simulink model "clean_SU_PEREHOD"  (R2021a)
settings: Solver=VariableStepAuto  StartTime=0.0  StopTime=stop  MaxStep=maxdt  MinStep=maxdt/10  RelTol=1e-5
values from neighbouring files (symbols this model uses):
  a_1P = M1U/J1K    (= 0.00153380423814)    [NASTROYKI.m]
  a_2P = M2U/J2K    (= 0.00155623811613)    [NASTROYKI.m]
  a_3P = M3U/J3K    (= 0.00948306595365)    [NASTROYKI.m]
  dt = 5    [NASTROYKI_STAB.m]
  DtR = pi/180    (= 0.0174532925199)    [NASTROYKI.m]    (also in NASTROYKI_STAB.m; NASTROYKI_VSEGO.m)
  g_1P = (M1B+Mmah)/J3K    (= 2.22905525847e-05)    [NASTROYKI.m]
  g_2P = (M2B+Mmah)/J3K    (= 2.22825311943e-05)    [NASTROYKI.m]
  g_3P = (M3B+Mmah)/J3K    (= 2.22905525847e-05)    [NASTROYKI.m]
  J2K = 6837    [NASTROYKI.m]    (also in NASTROYKI_STAB.m; NASTROYKI_VSEGO.m)
  J2M = 2    [NASTROYKI.m]    (also in NASTROYKI_STAB.m; NASTROYKI_VSEGO.m)
  k_1P = 0.5*sqrt((y_0_1P^2)/(2*a_1P^2*RtD^2))    [NASTROYKI.m]
  k_2P = 0.5*sqrt((y_0_2P^2)/(2*a_2P^2*RtD^2))    [NASTROYKI.m]
  k_3P = 0.5*sqrt((y_0_3P^2)/(2*a_3P^2*RtD^2))    [NASTROYKI.m]
  RtD = 1/DtR    (= 57.2957795131)    [NASTROYKI.m]    (also in NASTROYKI_STAB.m; NASTROYKI_VSEGO.m)
  x_0_1P = 0    [NASTROYKI.m]
  x_0_2P = 0    [NASTROYKI.m]
  x_0_3P = 0    [NASTROYKI.m]
  y_0_1P = a_1P*RtD*tmin/2*10    (= 0.00878805094449)    [NASTROYKI.m]
  y_0_2P = a_2P*RtD*tmin/2*10    (= 0.00891658759718)    [NASTROYKI.m]
  y_0_3P = a_3P*RtD*tmin/2*10    (= 0.0543339655989)    [NASTROYKI.m]
undefined symbols (not defined in the file or in its folder): Earth, WGS84
libraries: aerolibanim x4, templibrary x3, aerolibfltsims x2, aerolibtransform2 x1
settings Model: SimulationMode=rapid-accelerator  Creator=vanya  LastModifiedBy=vanya
settings SolverCC: MaxConsecutiveMinStep=50  ShapePreserveControl=EnableAll  ZeroCrossControl=DisableAll  ZeroCrossAlgorithm=Adaptive
settings DebuggingCC: IgnoredZcDiagnostic=none

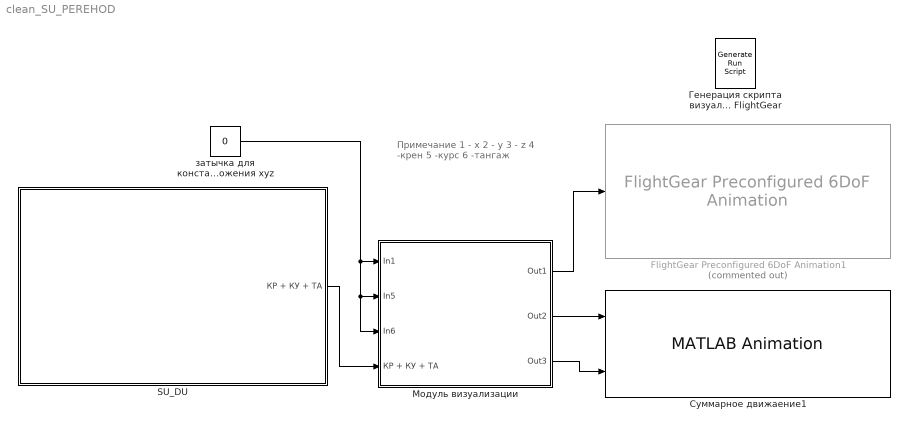
== system clean_SU_PEREHOD ==
  note: Примечание
      | 1 - x
      | 2 - y
      | 3 - z
      | 4 -крен
      | 5 -курс
      | 6 -тангаж
  FlightGear Preconfigured 6DoF Animation1 : aerolibfltsims/FlightGear Preconfigured 6DoF Animation  Commented=on  xFlightGearVersion=v2017.3  DestinationIpAddress=127.0.0.1  DestinationPort=5502  SampleTime=dt  packetVersion=24
  SU_DU : Subsystem
  Генерация скрипта визуализации в FlightGear : aerolibfltsims/Generate Run Script  Architecture=Default  dataFlow=Send  GeometryModelName=14bis  AirportId=KSFO  RunwayId=10L  InitialAltitude=722*100  InitialHeading=113  OffsetDistance=4.72  OffsetAzimuth=0  InstallScenery=off  DisableShaders=off  OriginAddress=127.0.0.1  DestinationPort=5502  OriginPort=5505  LocalAddress=127.0.0.1  OutputFileName=runfg.bat  FlightGearBaseDirectory=C:\Program Files\FlightGear 2020.3
  Модуль визуализации : Subsystem
  Суммарное движаение1 : aerolibanim/MATLAB Animation  Tag=Matlab Animation 6 DOF  Vehicles=1  Geometries='astredwedge.mat'  BoundingBoxCoordinates=[-50,50,-50,50,-50,50]  CameraOffset=[150,-150,-150]  CameraViewAngle=1  SampleTime=0.1  FigurePosition=[1,41,1920,990]
      settings: SourceProductBaseCode=AE
  затычка для константного положения xyz : Constant  Value=0
  wires:
  Модуль визуализации/2(Out2) -> Суммарное движаение1/1
  затычка для константного положения xyz/1 -> Модуль визуализации/3(In6), Модуль визуализации/2(In5), Модуль визуализации/1(In1)
  Модуль визуализации/1(Out1) -> FlightGear Preconfigured 6DoF Animation1/1
  SU_DU/1(КР + КУ + ТА) -> Модуль визуализации/4(КР + КУ + ТА)
  Модуль визуализации/3(Out3) -> Суммарное движаение1/2

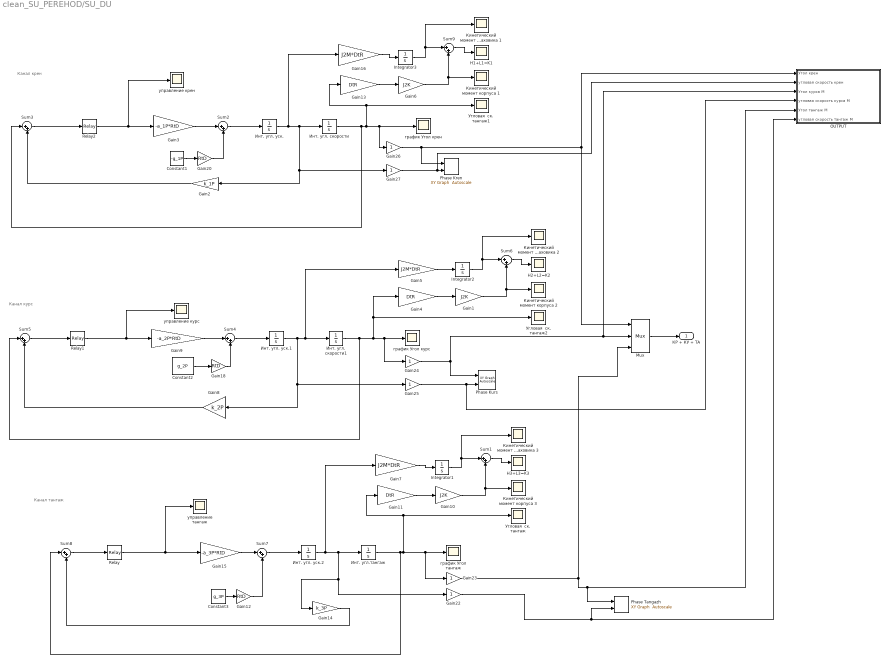
== system clean_SU_PEREHOD/SU_DU ==
  note: Канал крен
  note: Канал курс
  note: Канал тангаж
  " Кинетический момент корпуса 1" : Scope
  " Кинетический момент корпуса 2" : Scope
  " Кинетический момент корпуса 3" : Scope
  Constant1 : Constant  Value=-g_1P
  Constant2 : Constant  Value=g_2P
  Constant3 : Constant  Value=g_3P
  Gain1 : Gain  Gain=J2K
  Gain10 : Gain  Gain=J2K
  Gain11 : Gain  Gain=DtR
  Gain12 : Gain  Gain=RtD
  Gain13 : Gain  Gain=DtR
  Gain14 : Gain  Gain=k_3P
  Gain15 : Gain  Gain=-a_3P*RtD
  Gain16 : Gain  Gain=J2M*DtR
  Gain18 : Gain  Gain=RtD
  Gain2 : Gain  Gain=k_1P
  Gain20 : Gain  Gain=RtD
  Gain{22..27} (6 alike) : Gain
  Gain3 : Gain  Gain=-a_1P*RtD
  Gain4 : Gain  Gain=DtR
  Gain5 : Gain  Gain=J2M*DtR
  Gain6 : Gain  Gain=J2K
  Gain7 : Gain  Gain=J2M*DtR
  Gain8 : Gain  Gain=k_2P
  Gain9 : Gain  Gain=-a_2P*RtD
  H1+L1=K1 : Scope
  H2+L2=K2 : Scope
  H3+L3=K3 : Scope
  Integrator1 : Integrator
  Integrator2 : Integrator
  Integrator3 : Integrator
  Mux : Mux  Inputs=3
  OUTPUT : Subsystem
  Phase Kren : templibrary/XY Graph  Autoscale  xmin=-1  xmax=1  ymin=-1  ymax=1  st=-1
  Phase Kurs : templibrary/XY Graph  Autoscale  xmin=-1  xmax=1  ymin=-1  ymax=1  st=-1
  Phase Tangazh : templibrary/XY Graph  Autoscale  xmin=-1  xmax=1  ymin=-1  ymax=1  st=-1
  Relay : Relay  OnSwitchValue=0  OffSwitchValue=0  OffOutputValue=-1
  Relay1 : Relay  OnSwitchValue=0  OffSwitchValue=0  OffOutputValue=-1
  Relay2 : Relay  OnSwitchValue=0  OffSwitchValue=0  OffOutputValue=-1
  Sum{1..9} (9 alike) : Sum  Inputs=|++
  Инт. угл. скорости : Integrator  InitialCondition=x_0_1P
  Инт. угл. скорости1 : Integrator  InitialCondition=x_0_2P
  Инт. угл. уск. : Integrator  InitialCondition=y_0_1P
  Инт. угл. уск.1 : Integrator  InitialCondition=y_0_2P
  Инт. угл. уск.2 : Integrator  InitialCondition=y_0_3P
  Инт. угл.тангаж : Integrator  InitialCondition=x_0_3P
  Кинетический момент маховика 1 : Scope
  Кинетический момент маховика 2 : Scope
  Кинетический момент маховика 3 : Scope
  Угловая  ск. тангаж : Scope
  Угловая  ск. тангаж1 : Scope
  Угловая  ск. тангаж2 : Scope
  график Угол крен : Scope
  график Угол курс : Scope
  график Угол тангаж : Scope
  управление крен : Scope
  управление курс : Scope
  управление тангаж : Scope
  КР + КУ + ТА : Outport
  wires:
  Gain9/1 -> Sum4/1
  Gain2/1 -> Sum3/2
  Relay1/1 -> Gain9/1, управление курс/1
  Sum5/1 -> Relay1/1
  Sum2/1 -> Инт. угл. уск./1
  Gain15/1 -> Sum7/1
  Gain14/1 -> Sum8/2
  Sum8/1 -> Relay/1
  Gain3/1 -> Sum2/1
  Sum3/1 -> Relay2/1
  Sum4/1 -> Инт. угл. уск.1/1
  Gain8/1 -> Sum5/2
  Relay2/1 -> управление крен/1, Gain3/1
  Sum7/1 -> Инт. угл. уск.2/1
  Relay/1 -> управление тангаж/1, Gain15/1
  Constant3/1 -> Gain12/1
  Gain12/1 -> Sum7/2
  Constant2/1 -> Gain18/1
  Gain18/1 -> Sum4/2
  Constant1/1 -> Gain20/1
  Gain20/1 -> Sum2/2
  Mux/1 -> КР + КУ + ТА/1
  Инт. угл.тангаж/1 -> Угловая  ск. тангаж/1, Gain11/1, график Угол тангаж/1, Gain23/1, Sum8/1
  Gain7/1 -> Integrator1/1
  Инт. угл. уск.2/1 -> Gain7/1, Gain22/1, Gain14/1, Инт. угл.тангаж/1
  Gain11/1 -> Gain10/1
  Integrator1/1 -> Кинетический момент маховика 3/1, Sum1/1
  Gain10/1 -> " Кинетический момент корпуса 3"/1, Sum1/2
  Sum1/1 -> H3+L3=K3/1
  Sum6/1 -> H2+L2=K2/1
  Gain4/1 -> Gain1/1
  Integrator2/1 -> Кинетический момент маховика 2/1, Sum6/1
  Инт. угл. скорости1/1 -> Угловая  ск. тангаж2/1, Gain4/1, график Угол курс/1, Gain24/1, Sum5/1
  Gain5/1 -> Integrator2/1
  Инт. угл. уск.1/1 -> Gain5/1, Инт. угл. скорости1/1, Gain25/1, Gain8/1
  Gain1/1 -> " Кинетический момент корпуса 2"/1, Sum6/2
  Sum9/1 -> H1+L1=K1/1
  Gain13/1 -> Gain6/1
  Integrator3/1 -> Кинетический момент маховика 1/1, Sum9/1
  Инт. угл. скорости/1 -> Угловая  ск. тангаж1/1, Gain13/1, Gain26/1, график Угол крен/1, Sum3/1
  Gain16/1 -> Integrator3/1
  Инт. угл. уск./1 -> Gain16/1, Gain27/1, Gain2/1, Инт. угл. скорости/1
  Gain6/1 -> " Кинетический момент корпуса 1"/1, Sum9/2
  Gain25/1 -> OUTPUT/4(угловая скорость курса М), Phase Kurs/2
  Gain22/1 -> OUTPUT/6(угловая скорость тангаж М), Phase Tangazh/2
  Gain27/1 -> OUTPUT/2(угловая скорость крен), Phase Kren/2
  Gain26/1 -> Phase Kren/1, OUTPUT/1(Угол крен), Mux/1
  Gain24/1 -> OUTPUT/3(Угол курса М), Mux/2, Phase Kurs/1
  Gain23/1 -> Mux/3, OUTPUT/5(Угол тангаж М), Phase Tangazh/1

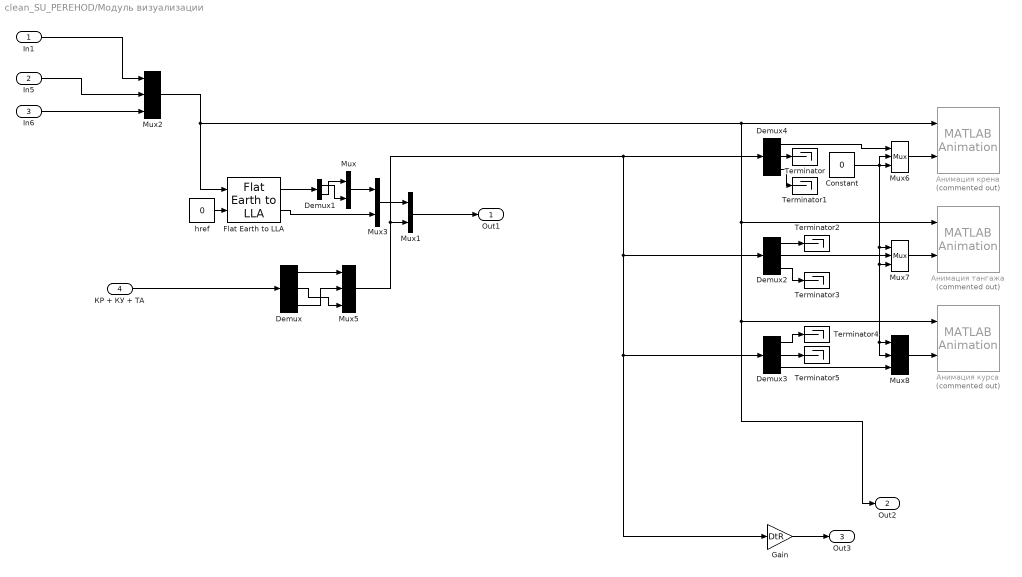
== system clean_SU_PEREHOD/Модуль визуализации ==
  In1 : Inport
  In5 : Inport  Port=2
  In6 : Inport  Port=3
  КР + КУ + ТА : Inport  Port=4
  Constant : Constant  Value=0
  Demux{,2..4} (4 alike) : Demux  Outputs=3
  Demux1 : Demux  Outputs=2
  Flat Earth to LLA : aerolibtransform2/Flat Earth to LLA  units=Metric (MKS)  ptype=Earth (WGS84)  F=1/298.257223563  R=6378137  refPosPort=off  LL0=[37.61 -122.39]  psi=0
  Gain : Gain  Gain=DtR
  Mux : Mux  Inputs=2
  Mux1 : Mux  Inputs=2
  Mux{2,5..8} (5 alike) : Mux  Inputs=3
  Mux3 : Mux  Inputs=2
  Terminator{,1..5} (6 alike) : Terminator
  href : Constant  Value=0
  Анимация крена : aerolibanim/MATLAB Animation  Tag=Matlab Animation 6 DOF  Commented=on  Vehicles=1  Geometries='astredwedge.mat'  BoundingBoxCoordinates=[-50,50,-50,50,-50,50]  CameraOffset=[-50,-50,-50]  CameraViewAngle=2  SampleTime=0.2  FigurePosition=[786,232,729,287]
      settings: SourceProductBaseCode=AE
  Анимация курса : aerolibanim/MATLAB Animation  Tag=Matlab Animation 6 DOF  Commented=on  Vehicles=1  Geometries='astredwedge.mat'  BoundingBoxCoordinates=[-50,50,-50,50,-50,50]  CameraOffset=[0,0,-400]  CameraViewAngle=1  SampleTime=0.2  FigurePosition=[529,247,612,404]
      settings: SourceProductBaseCode=AE
  Анимация тангажа : aerolibanim/MATLAB Animation  Tag=Matlab Animation 6 DOF  Commented=on  Vehicles=1  Geometries='astredwedge.mat'  BoundingBoxCoordinates=[-50,50,-50,50,-50,50]  CameraOffset=[-50,-50,-50]  CameraViewAngle=2  SampleTime=0.2  FigurePosition=[447,306,729,287]
      settings: SourceProductBaseCode=AE
  Out1 : Outport
  Out2 : Outport  Port=2
  Out3 : Outport  Port=3
  wires:
  Demux1/2 -> Mux/1
  КР + КУ + ТА/1 -> Demux/1
  Flat Earth to LLA/1 -> Demux1/1
  Mux/1 -> Mux3/1
  Mux3/1 -> Mux1/1
  href/1 -> Flat Earth to LLA/2
  Flat Earth to LLA/2 -> Mux3/2
  Mux1/1 -> Out1/1
  Demux1/1 -> Mux/2
  In1/1 -> Mux2/1
  In5/1 -> Mux2/2
  In6/1 -> Mux2/3
  Demux4/3 -> Terminator1/1
  Demux3/1 -> Terminator4/1
  Mux7/1 -> Анимация тангажа/2
  Demux3/2 -> Terminator5/1
  Demux2/1 -> Terminator2/1
  Demux2/2 -> Mux7/2
  Mux6/1 -> Анимация крена/2
  Demux3/3 -> Mux8/3
  Demux4/2 -> Terminator/1
  Constant/1 -> Mux7/3, Mux8/2, Mux8/1, Mux7/1, Mux6/2, Mux6/3
  Demux4/1 -> Mux6/1
  Mux8/1 -> Анимация курса/2
  Demux2/3 -> Terminator3/1
  Mux2/1 -> Анимация крена/1, Анимация тангажа/1, Анимация курса/1, Out2/1, Flat Earth to LLA/1
  Mux5/1 -> Demux4/1, Demux2/1, Gain/1, Demux3/1, Mux1/2
  Demux/1 -> Mux5/1
  Demux/3 -> Mux5/2
  Demux/2 -> Mux5/3
  Gain/1 -> Out3/1

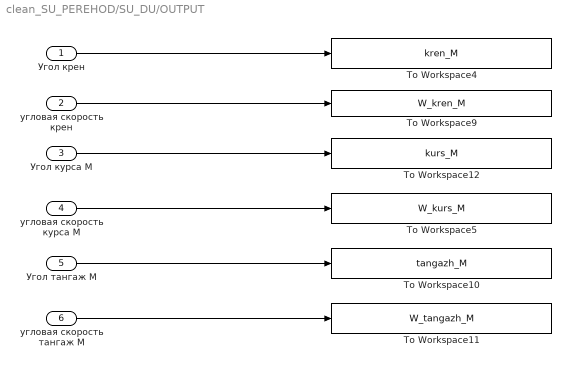
== system clean_SU_PEREHOD/SU_DU/OUTPUT ==
  Угол крен : Inport
  угловая скорость крен : Inport  Port=2
  Угол курса М : Inport  Port=3
  угловая скорость курса М : Inport  Port=4
  Угол тангаж М : Inport  Port=5
  угловая скорость тангаж М : Inport  Port=6
  To Workspace10 : ToWorkspace  VariableName=tangazh_M  SampleTime=-1
      settings: Save2DSignal=2-D array (concatenate along first dimension)
  To Workspace11 : ToWorkspace  VariableName=W_tangazh_M  SampleTime=-1
      settings: Save2DSignal=2-D array (concatenate along first dimension)
  To Workspace12 : ToWorkspace  VariableName=kurs_M  SampleTime=-1
      settings: Save2DSignal=2-D array (concatenate along first dimension)
  To Workspace4 : ToWorkspace  VariableName=kren_M  SampleTime=-1
      settings: Save2DSignal=2-D array (concatenate along first dimension)
  To Workspace5 : ToWorkspace  VariableName=W_kurs_M  SampleTime=-1
      settings: Save2DSignal=2-D array (concatenate along first dimension)
  To Workspace9 : ToWorkspace  VariableName=W_kren_M  SampleTime=-1
      settings: Save2DSignal=2-D array (concatenate along first dimension)
  wires:
  Угол курса М/1 -> To Workspace12/1
  угловая скорость крен/1 -> To Workspace9/1
  угловая скорость курса М/1 -> To Workspace5/1
  угловая скорость тангаж М/1 -> To Workspace11/1
  Угол крен/1 -> To Workspace4/1
  Угол тангаж М/1 -> To Workspace10/1
